simulink model "sim_LQI"  (R2016a)
settings: Solver=VariableStepAuto  StartTime=0.0  StopTime=180  RelTol=1e-3
undefined symbols (not defined in the file or in its folder): Continuous, K, sys, Time
libraries: simulink x2, ctrlSharedLib x1, lib_Lagrangian_Model_Nonlinear x1
settings Model: Creator=ottoe  LastModifiedBy=ottoe

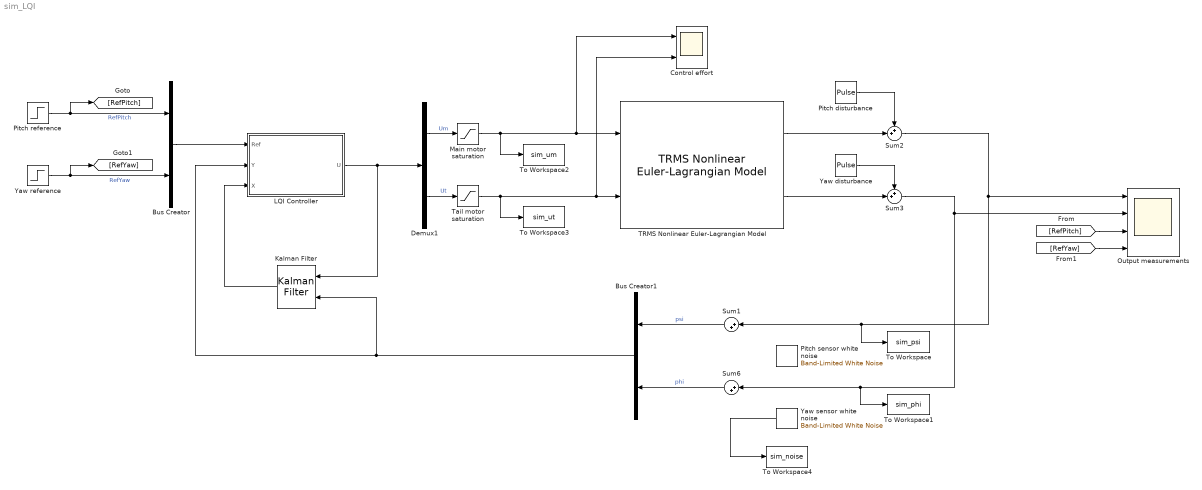
== system sim_LQI ==
  Bus Creator : BusCreator  Inputs=2
  Bus Creator1 : BusCreator  Inputs=2
  Control effort : Scope  NumInputPorts=2
  Demux1 : Demux  Outputs=2
  Kalman Filter : ctrlSharedLib/Kalman Filter  TimeDomain=Continuous-Time  UseCurrentEstimator=on  ModelSource=Individual A, B, C, D matrices  ModelSourceVariable=ss(0.95,1,1,0,1)  A=sys.A  B=sys.B  C=sys.C  D=sys.D  NumberOfStates=1  NumberOfInputs=1  NumberOfOutputs=1  InitialEstimateSource=Dialog  X0=[0 0 0 0 0 0]'  P0=10  UseK=off  UseGH=off  NumberOfProcessNoiseInputs=1  G=1  TimeInvariantG=on  H=0  TimeInvariantH=on  Q=1000  TimeInvariantQ=on  R=0.1  TimeInvariantR=on  N=0  TimeInvariantN=on  AddInputPort=on  AddEnablePort=off  ExternalReset=none  OutputEstimatedY=off  OutputP=off  Ts=-1
  LQI Controller : Subsystem
  Main motor saturation : Saturate  UpperLimit=2.5  LowerLimit=-2.5
  Output measurements : Scope  NumInputPorts=4
  Pitch disturbance : DiscretePulseGenerator  PulseType=Time based  Amplitude=0.1  Period=100  PulseWidth=0.1  PhaseDelay=80
  Pitch reference : Step  Time=100  After=0  SampleTime=0
  Pitch sensor white noise : simulink/Sources/Band-Limited White Noise  Cov=[0.000000001]  Ts=0.001  seed=[23341]
  Sum1 : Sum  Inputs=|++
  Sum2 : Sum  Inputs=++|
  Sum3 : Sum  Inputs=++|
  Sum6 : Sum  Inputs=|++
  TRMS Nonlinear Euler-Lagrangian Model : lib_Lagrangian_Model_Nonlinear/TRMS Nonlinear Euler-Lagrangian Model  Psi_zero=0  Psi_dot_zero=0  Phi_zero=0  Phi_dot_zero=0  Wm_zero=0  Wt_zero=0
  Tail motor saturation : Saturate  UpperLimit=2.5  LowerLimit=-2.5
  To Workspace : ToWorkspace  VariableName=sim_psi  SaveFormat=Timeseries  SampleTime=-1
  To Workspace1 : ToWorkspace  VariableName=sim_phi  SaveFormat=Timeseries  SampleTime=-1
  To Workspace2 : ToWorkspace  VariableName=sim_um  SaveFormat=Timeseries  SampleTime=-1
  To Workspace3 : ToWorkspace  VariableName=sim_ut  SaveFormat=Timeseries  SampleTime=-1
  To Workspace4 : ToWorkspace  VariableName=sim_noise  SaveFormat=Timeseries  SampleTime=-1
  Yaw disturbance : DiscretePulseGenerator  PulseType=Time based  Amplitude=0.1  Period=100  PulseWidth=0.1  PhaseDelay=120
  Yaw reference : Step  Time=140  After=0  SampleTime=0
  Yaw sensor white noise : simulink/Sources/Band-Limited White Noise  Cov=[0.000000001]  Ts=0.001  seed=[23341]
  wires:
  Pitch reference/1 -> [RefPitch], Bus Creator/1  "RefPitch"
  Yaw reference/1 -> [RefYaw], Bus Creator/2  "RefYaw"
  TRMS Nonlinear Euler-Lagrangian Model/1 -> Sum2/2
  TRMS Nonlinear Euler-Lagrangian Model/2 -> Sum3/2
  Pitch disturbance/1 -> Sum2/1
  Yaw disturbance/1 -> Sum3/1
  Sum3/1 -> Output measurements/2, To Workspace1/1, Sum6/1
  Sum2/1 -> Output measurements/1, To Workspace/1, Sum1/1
  [RefPitch] -> Output measurements/3
  [RefYaw] -> Output measurements/4
  Demux1/2 -> Tail motor saturation/1  "Ut"
  Demux1/1 -> Main motor saturation/1  "Um"
  Main motor saturation/1 -> To Workspace2/1, Control effort/1, TRMS Nonlinear Euler-Lagrangian Model/1
  Tail motor saturation/1 -> To Workspace3/1, Control effort/2, TRMS Nonlinear Euler-Lagrangian Model/2
  LQI Controller/1(U) -> Kalman Filter/1, Demux1/1
  Kalman Filter/1 -> LQI Controller/3(X)
  Bus Creator/1 -> LQI Controller/1(Ref)
  Bus Creator1/1 -> Kalman Filter/2, LQI Controller/2(Y)
  Yaw sensor white noise/1 -> To Workspace4/1
  Sum1/1 -> Bus Creator1/1  "psi"
  Sum6/1 -> Bus Creator1/2  "phi"

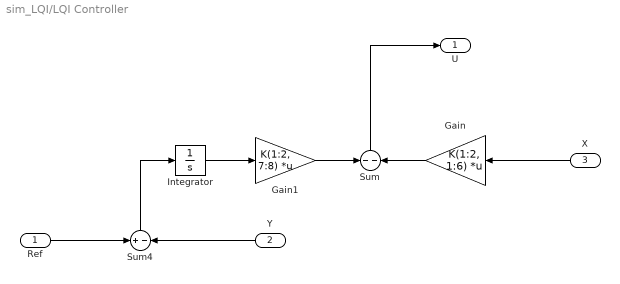
== system sim_LQI/LQI Controller ==
  Ref : Inport
  Y : Inport  Port=2
  X : Inport  Port=3
  Gain : Gain  Gain=K(1:2, 1:6)  Multiplication=Matrix(K*u) (u vector)
  Gain1 : Gain  Gain=K(1:2, 7:8)  Multiplication=Matrix(K*u) (u vector)
  Integrator : Integrator  InitialCondition=[0, 0]
  Sum : Sum  Inputs=-|-
  Sum4 : Sum  Inputs=+|-
  U : Outport
  wires:
  X/1 -> Gain/1
  Integrator/1 -> Gain1/1
  Ref/1 -> Sum4/1
  Y/1 -> Sum4/2
  Gain/1 -> Sum/2
  Sum/1 -> U/1
  Gain1/1 -> Sum/1
  Sum4/1 -> Integrator/1
